simulink model "PFE_2Lignes_RNA (2)"  (R2024a)
settings: Solver=ode4  StartTime=0.0  StopTime=0.18  RelTol=1e-3
libraries: neural x202, spsRMSLib x12, spsThreePhasePISectionLineLib x4, spsThreePhaseFaultLib x2, spsThreePhaseVIMeasurementLib x2, spsThreePhaseSourceLib x2, spspowerguiLib x1
(part 10 of 10)

== system PFE_2Lignes_RNA (2)/RNA_Localisateur/Layer 3/Delays 1 ==
  "p{3}" : Inport  PortDimensions=25
      mask Display: e = 0.06;c1 = [120 230 180]/255;c2 = ([120 230 180]+0)/(256+128);c3 = ([120 230 180]+128)/(256+128);patch([0 1 1 0],[0 0 1 1],c1);patch([0 1 1 1-e 1-e 0+e],[0 0 1 1-e 0+e 0+e],c2);patch([0 0 1 1-e 0+e 0+e],[0 1 1 1-e 1-e 0+e],c3);plot([0 1 1 0 0],[0 0 1 1 0]);
  mux : Mux  Inputs=1
      mask Display: e = 0.06;c1 = [120 150 230]/255;c2 = ([120 150 230]+0)/383;c3 = ([120 150 230]+128)/383;patch([0 1 1 0],[0 0 1 1],c1);patch([0 1 1 1-e 1-e 0+e],[0 0 1 1-e 0+e 0+e],c2);patch([0 0 1 1-e 0+e 0+e],[0 1 1 1-e 1-e 0+e],c3);plot([0 1 1 0 0],[0 0 1 1 0]);disp('Mux')
  "pd{3,2}" : Outport
      mask Display: e = 0.06;c1 = [120 230 180]/255;c2 = ([120 230 180]+0)/(256+128);c3 = ([120 230 180]+128)/(256+128);patch([0 1 1 0],[0 0 1 1],c1);patch([0 1 1 1-e 1-e 0+e],[0 0 1 1-e 0+e 0+e],c2);patch([0 0 1 1-e 0+e 0+e],[0 1 1 1-e 1-e 0+e],c3);plot([0 1 1 0 0],[0 0 1 1 0]);
  wires:
  "p{3}"/1 -> mux/1
  mux/1 -> "pd{3,2}"/1

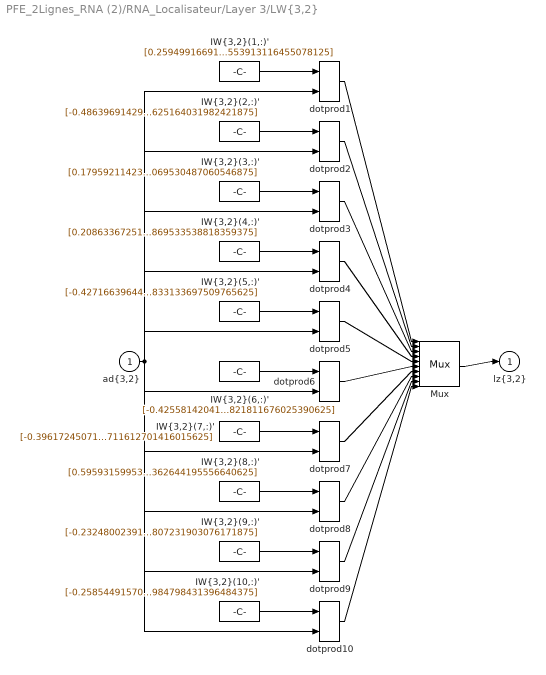
== system PFE_2Lignes_RNA (2)/RNA_Localisateur/Layer 3/LW{3,2} ==
  "ad{3,2}" : Inport  PortDimensions=25
      mask Display: e = 0.06;c1 = [120 230 180]/255;c2 = ([120 230 180]+0)/(256+128);c3 = ([120 230 180]+128)/(256+128);patch([0 1 1 0],[0 0 1 1],c1);patch([0 1 1 1-e 1-e 0+e],[0 0 1 1-e 0+e 0+e],c2);patch([0 0 1 1-e 0+e 0+e],[0 1 1 1-e 1-e 0+e],c3);plot([0 1 1 0 0],[0 0 1 1 0]);
  "IW{3,2}(1,:)'" : Constant  Value=[0.259499166914273715622840654759784229099750518798828125;-0.257383375091483734831143692645127885043621063232421875;-0.0215920617215718847747840669626384624280035495758056640625;-0.38639212006215284400667542286100797355175018310546875;0.0724580935613540477735483591459342278540134429931640625;-0.153650430968274964715902797252056188881397247314453125;-0.5162510887242304224997724304557777941226959228515625;0.0225239402589197008908161734552777488715946674346923828125;-0.330358684113883527277977236735750921070575714111328125;0.169424344213606470344046783793601207435131072998046875;0.07892490230528238781548822089462191797792911529541015625;0.8200359869986921790285805400344543159008026123046875;0.124512774480091514828217214017058722674846649169921875;0.1442480998551381732308840355472057126462459564208984375;-0.53065073451970057316628981425310485064983367919921875;0.2116724722061891217350648730644024908542633056640625;0.16550316479374627132159503162256442010402679443359375;0.396942477917246849816734766136505641043186187744140625;0.033487838311827382298258015680403332225978374481201171875;-0.2078927394991537946911108747372054494917392730712890625;0.24309155258077008721073752894881181418895721435546875;0.2102599726857405648683396748310769908130168914794921875;0.28148895042717192449543972543324343860149383544921875;0.15969935949450875245503311816719360649585723876953125;-0.4549152584406943589101501856930553913116455078125]
      mask Display: e = 0.06;c1 = [120 150 230]/255;c2 = ([120 150 230]+0)/383;c3 = ([120 150 230]+128)/383;patch([0 1 1 0],[0 0 1 1],c1);patch([0 1 1 1-e 1-e 0+e],[0 0 1 1-e 0+e 0+e],c2);patch([0 0 1 1-e 0+e 0+e],[0 1 1 1-e 1-e 0+e],c3);plot([0 1 1 0 0],[0 0 1 1 0]);disp('weights');
  "IW{3,2}(10,:)'" : Constant  Value=[-0.25854491570469650962849073039251379668712615966796875;0.196184940707442134755211782248807139694690704345703125;0.7645250944377817159391952372970990836620330810546875;-0.0184527315099401560682945699909396353177726268768310546875;0.367147579101182841565531589367310516536235809326171875;0.331249780882799382819570155334076844155788421630859375;0.3277245040461982394930373629904352128505706787109375;-0.253855352684368040794282705974183045327663421630859375;0.29341155210540825759579774967278353869915008544921875;0.08151026931019385302068513965423335321247577667236328125;0.1810431757750518844130027673600125126540660858154296875;0.2314159756638828613350966634243377484381198883056640625;0.08787736385978257847018113579906639643013477325439453125;-0.37698257865251705300835283196647651493549346923828125;0.315315557570428506295456827501766383647918701171875;0.33180976505799197884272189185139723122119903564453125;-0.25777939796702875607792293521924875676631927490234375;0.79791774501736811853191966292797587811946868896484375;-0.59432999568261346556852231515222229063510894775390625;-0.61707616054659808479954108406673185527324676513671875;-0.730705022070508025677781915874220430850982666015625;-0.360402877050402137282247849725536070764064788818359375;-0.36782434924704343615076140849851071834564208984375;-0.260230331044378926375060245845816098153591156005859375;-0.27207637131283080034194199470221064984798431396484375]
      mask Display: e = 0.06;c1 = [120 150 230]/255;c2 = ([120 150 230]+0)/383;c3 = ([120 150 230]+128)/383;patch([0 1 1 0],[0 0 1 1],c1);patch([0 1 1 1-e 1-e 0+e],[0 0 1 1-e 0+e 0+e],c2);patch([0 0 1 1-e 0+e 0+e],[0 1 1 1-e 1-e 0+e],c3);plot([0 1 1 0 0],[0 0 1 1 0]);disp('weights');
  "IW{3,2}(2,:)'" : Constant  Value=[-0.486396914294387971988697927372413687407970428466796875;-0.2992436697012557100805452137137763202190399169921875;-1.0096640245988937056864642727305181324481964111328125;-0.7633555721722729003886342979967594146728515625;0.319862500795322912683360527807963080704212188720703125;-0.1381707631856110840562479324944433756172657012939453125;0.05730667196484000303069450410475837998092174530029296875;0.60670341083743528631799790673539973795413970947265625;0.162744168043399473067012195315328426659107208251953125;0.76390045801718053919415751806809566915035247802734375;-0.251036863009820365721935786496032960712909698486328125;0.348548775645059760730504194725654087960720062255859375;-1.2651758025279082886527248774655163288116455078125;0.5701608488095846194454452415811829268932342529296875;-0.45746006806566763547294840464019216597080230712890625;0.1775172818765219096004415177958435378968715667724609375;0.83109712322488393798636252540745772421360015869140625;-0.002819460130945704127991557896848462405614554882049560546875;-1.3113587123974017600858132936991751194000244140625;-0.94794595241073997815561824609176255762577056884765625;-0.8672272284534410236034318586462177336215972900390625;0.31406958478618396402026746727642603218555450439453125;-0.66306336271592503095462234341539442539215087890625;0.70909112904029758528423599273082800209522247314453125;-0.1927834405910741899514704300599987618625164031982421875]
      mask Display: e = 0.06;c1 = [120 150 230]/255;c2 = ([120 150 230]+0)/383;c3 = ([120 150 230]+128)/383;patch([0 1 1 0],[0 0 1 1],c1);patch([0 1 1 1-e 1-e 0+e],[0 0 1 1-e 0+e 0+e],c2);patch([0 0 1 1-e 0+e 0+e],[0 1 1 1-e 1-e 0+e],c3);plot([0 1 1 0 0],[0 0 1 1 0]);disp('weights');
  "IW{3,2}(3,:)'" : Constant  Value=[0.1795921142321371399841467564328922890126705169677734375;-0.0830058214984936981739593875317950733006000518798828125;0.42600710957444254400883210109896026551723480224609375;0.56216901247103800987048316528671421110630035400390625;0.214484010219940568475749387289397418498992919921875;0.65506656139687013951089511465397663414478302001953125;-0.2738986952750577241744167622528038918972015380859375;-0.40274361448586504241831107719917781651020050048828125;0.75469640022346806684794273678562603890895843505859375;0.16066872870166559739146805441123433411121368408203125;0.4675408868247641347437593140057288110256195068359375;0.339255842745214142297527359914965927600860595703125;-0.76204632162776364534551021279185079038143157958984375;0.411196253292331892481570321251638233661651611328125;-0.37118321250245944753487492562271654605865478515625;-0.34219671096980908142626276458031497895717620849609375;-0.26652835547218012290926481000497005879878997802734375;0.46914434545171557200404777177027426660060882568359375;-0.2265549344525312758236168519943021237850189208984375;-0.250327500477882713969535188880399800837039947509765625;-0.5644921592451357383879440021701157093048095703125;-0.02543337437470427619956581111182458698749542236328125;0.215714533272492403614961631319602020084857940673828125;0.133709939839643354719811441100318916141986846923828125;0.45080169671964920308226965062203817069530487060546875]
      mask Display: e = 0.06;c1 = [120 150 230]/255;c2 = ([120 150 230]+0)/383;c3 = ([120 150 230]+128)/383;patch([0 1 1 0],[0 0 1 1],c1);patch([0 1 1 1-e 1-e 0+e],[0 0 1 1-e 0+e 0+e],c2);patch([0 0 1 1-e 0+e 0+e],[0 1 1 1-e 1-e 0+e],c3);plot([0 1 1 0 0],[0 0 1 1 0]);disp('weights');
  "IW{3,2}(4,:)'" : Constant  Value=[0.208633672511950918337930716006667353212833404541015625;-0.049774452361300458580473105030250735580921173095703125;0.439326907042213388177032129533472470939159393310546875;0.171290457666205264697367738335742615163326263427734375;0.540872208754529015806156166945584118366241455078125;-0.2331890730032175340635802740507642738521099090576171875;-0.46194631852841505637030650177621282637119293212890625;0.354039924065002786779388088689302094280719757080078125;0.48242957728458579769181824303814209997653961181640625;0.7025339975202451459068697658949531614780426025390625;-0.471942860262994423603544191792025230824947357177734375;-0.34067847690385588688144480329356156289577484130859375;-0.10191518091187268257868936416343785822391510009765625;0.89719408490654384280560407205484807491302490234375;-0.1476056157321989636965753334152395837008953094482421875;0.371494341788785431557329275165102444589138031005859375;0.53142307222104723241073997996863909065723419189453125;-0.86911676430513173929881531876162625849246978759765625;0.95899584831374007354298782956902869045734405517578125;0.01514824633352983285217163711422472260892391204833984375;-0.0309472140695323354175894081663500401191413402557373046875;0.0227440549634588227989606679102507769130170345306396484375;0.2054332578510936480054027697406127117574214935302734375;0.47578074684271276506564163355506025254726409912109375;-0.493126298182259004132532709263614378869533538818359375]
      mask Display: e = 0.06;c1 = [120 150 230]/255;c2 = ([120 150 230]+0)/383;c3 = ([120 150 230]+128)/383;patch([0 1 1 0],[0 0 1 1],c1);patch([0 1 1 1-e 1-e 0+e],[0 0 1 1-e 0+e 0+e],c2);patch([0 0 1 1-e 0+e 0+e],[0 1 1 1-e 1-e 0+e],c3);plot([0 1 1 0 0],[0 0 1 1 0]);disp('weights');
  "IW{3,2}(5,:)'" : Constant  Value=[-0.42716639644105691697717475108220241963863372802734375;0.319735122611505107048657237100997008383274078369140625;-0.144913256802170875570112684727064333856105804443359375;0.418094711227112558749041681949165649712085723876953125;0.511325541048309961666973322280682623386383056640625;-0.008907182515639870679091671945570851676166057586669921875;-0.289029559077883357876004311037831939756870269775390625;-0.01209733468703781157638221799288658075965940952301025390625;0.039414040601209114622616169754110160283744335174560546875;-0.08724077377198026506111006028731935657560825347900390625;0.93062461612003410937887792897527106106281280517578125;-0.84348086792044563164694181978120468556880950927734375;-0.33012975187102266971805875073187053203582763671875;0.6052379701685082213913347004563547670841217041015625;-0.59579112157312319464352867726120166480541229248046875;0.4111185993323529519472003812552429735660552978515625;0.45409004664972230091990468281437642872333526611328125;0.8687099235218556092519293088116683065891265869140625;0.35767499887355003185263058185228146612644195556640625;-0.59731612138546619217294164627674035727977752685546875;0.162670883357776741018341226663324050605297088623046875;-0.2230248190546767206310363462762325070798397064208984375;-0.573880672304131422833961551077663898468017578125;-0.45711823783840788149035461174207739531993865966796875;0.1625955550529826487693441094961599446833133697509765625]
      mask Display: e = 0.06;c1 = [120 150 230]/255;c2 = ([120 150 230]+0)/383;c3 = ([120 150 230]+128)/383;patch([0 1 1 0],[0 0 1 1],c1);patch([0 1 1 1-e 1-e 0+e],[0 0 1 1-e 0+e 0+e],c2);patch([0 0 1 1-e 0+e 0+e],[0 1 1 1-e 1-e 0+e],c3);plot([0 1 1 0 0],[0 0 1 1 0]);disp('weights');
  "IW{3,2}(6,:)'" : Constant  Value=[-0.425581420418537137440040396541007794439792633056640625;0.11336041614642834718384989400874474085867404937744140625;-0.293111819207529544772938834285014308989048004150390625;0.39126271714747107299814388170489110052585601806640625;0.44854646393908093049418539521866478025913238525390625;0.463505961310431591204661572191980667412281036376953125;-0.397849466360224834904357749110204167664051055908203125;0.284078924760211515287977590560331009328365325927734375;-0.414256591580237032435007904496160335838794708251953125;-0.374072668830715271415243705632747150957584381103515625;0.85195121714305976912129381162230856716632843017578125;0.06469055391895263407153748858036124147474765777587890625;0.85097433591525073470762663419009186327457427978515625;-0.181106906938278466867586757871322333812713623046875;0.34245989875019022807833835031487978994846343994140625;0.646702640754573732095877858228050172328948974609375;-0.5654784119053679614097518424387089908123016357421875;-0.36053840646464208052890398903400637209415435791015625;0.07719239096012538159374827273495611734688282012939453125;-0.28537380618497187878546128558809868991374969482421875;0.54880359654620658460544291301630437374114990234375;0.32469019193151826829790707051870413124561309814453125;0.246685178608404609423843112381291575729846954345703125;-0.2522084322168911540984481689520180225372314453125;0.057301412441833933508750220653382712043821811676025390625]
      mask Display: e = 0.06;c1 = [120 150 230]/255;c2 = ([120 150 230]+0)/383;c3 = ([120 150 230]+128)/383;patch([0 1 1 0],[0 0 1 1],c1);patch([0 1 1 1-e 1-e 0+e],[0 0 1 1-e 0+e 0+e],c2);patch([0 0 1 1-e 0+e 0+e],[0 1 1 1-e 1-e 0+e],c3);plot([0 1 1 0 0],[0 0 1 1 0]);disp('weights');
  "IW{3,2}(7,:)'" : Constant  Value=[-0.3961724507194579469882000921643339097499847412109375;0.1387250010604408612113758181294542737305164337158203125;0.79843909814126001744938321280642412602901458740234375;-0.13197386480330586255860225719516165554523468017578125;-0.963138474221520990425915442756377160549163818359375;0.77614602963594558904247833197587169706821441650390625;0.0459985084465074633985892660348326899111270904541015625;-0.32747154753047247321973145517404191195964813232421875;0.329878955635281745362163974277791567146778106689453125;-0.68783651058276207290731463217525742948055267333984375;1.7187260561734889474649889962165616452693939208984375;0.277645949269099745482236585303326137363910675048828125;-0.0973489866815408222411321048639365471899509429931640625;-1.09730793256456049533653640537522733211517333984375;0.478189280833778929125088552609668113291263580322265625;0.23624340435405011273672926108702085912227630615234375;-0.376796535196192439176599009442725218832492828369140625;0.89917669709510317233025489258579909801483154296875;-0.38151855174703774853384175003156997263431549072265625;-0.243324845860096450333998063797480426728725433349609375;-0.58220435207547371891934062659856863319873809814453125;0.2166088158148688214144073072020546533167362213134765625;0.667135572700811252389030414633452892303466796875;-0.77032076667743165643287284183315932750701904296875;0.036010859707251409445039058709880919195711612701416015625]
      mask Display: e = 0.06;c1 = [120 150 230]/255;c2 = ([120 150 230]+0)/383;c3 = ([120 150 230]+128)/383;patch([0 1 1 0],[0 0 1 1],c1);patch([0 1 1 1-e 1-e 0+e],[0 0 1 1-e 0+e 0+e],c2);patch([0 0 1 1-e 0+e 0+e],[0 1 1 1-e 1-e 0+e],c3);plot([0 1 1 0 0],[0 0 1 1 0]);disp('weights');
  "IW{3,2}(8,:)'" : Constant  Value=[0.5959315995396183840426829192438162863254547119140625;-0.68920983699735038907618900339002721011638641357421875;-0.547275052350105095655408149468712508678436279296875;-0.46668802981562673704019061915460042655467987060546875;0.70348097684159427434025246839155443012714385986328125;1.2358100589287006609851005123346112668514251708984375;-0.057695062285977379012980037487068329937756061553955078125;1.3383434388428316896835212901351042091846466064453125;0.95131380634382989303077238218975253403186798095703125;0.1426293234011531685379026157534099183976650238037109375;-0.54812770381903674898893541467259638011455535888671875;0.7382984438201518617717056258697994053363800048828125;-1.133045117712822236200054248911328613758087158203125;-0.94071248542285046401190129472524859011173248291015625;-0.222026415195621662501679338674875907599925994873046875;0.2989728874563242211337410481064580380916595458984375;0.80555562586803730606987983264843933284282684326171875;-1.630533738843426672104897079407237470149993896484375;-0.9069177750597390286202426068484783172607421875;-0.564683822516274691594162504770793020725250244140625;0.143682760802573195046960563558968715369701385498046875;1.4286546216244477847112648305483162403106689453125;-0.036125095413979291247841274525853805243968963623046875;0.354152440418581349046434070260147564113140106201171875;0.2022263960100302571110120197772630490362644195556640625]
      mask Display: e = 0.06;c1 = [120 150 230]/255;c2 = ([120 150 230]+0)/383;c3 = ([120 150 230]+128)/383;patch([0 1 1 0],[0 0 1 1],c1);patch([0 1 1 1-e 1-e 0+e],[0 0 1 1-e 0+e 0+e],c2);patch([0 0 1 1-e 0+e 0+e],[0 1 1 1-e 1-e 0+e],c3);plot([0 1 1 0 0],[0 0 1 1 0]);disp('weights');
  "IW{3,2}(9,:)'" : Constant  Value=[-0.232480023916576072906536865048110485076904296875;-0.164443579735376654848977295841905288398265838623046875;1.4179787649137292060430581841501407325267791748046875;0.25143330694485344078970001646666787564754486083984375;-0.510136233004576222782588956761173903942108154296875;-0.686297218738918246572211501188576221466064453125;-0.262326282237484331716359520214609801769256591796875;-0.597869214900524692524186320952139794826507568359375;-1.0275285597316126118272450185031630098819732666015625;-0.315286007568047532689803347238921560347080230712890625;0.393766399328244809385779490185086615383625030517578125;-0.5387605194849260925593625870533287525177001953125;-0.006413070897718455010139138039448880590498447418212890625;-0.45177115742190421254775856141350232064723968505859375;0.07537030025988909753831279658697894774377346038818359375;-0.9771504767164269633639150924864225089550018310546875;-0.261093310200134709475605632178485393524169921875;0.481535901719132131137968144685146398842334747314453125;0.570459672953978813580988571629859507083892822265625;0.181741283610712012208665555590414442121982574462890625;-0.79097702615542575532714408836909569799900054931640625;-0.0656079654481984686498208247940056025981903076171875;-0.6737649753269134844657628491404466331005096435546875;0.78476774835336005065045128503697924315929412841796875;-0.078997850155492599366624517642776481807231903076171875]
      mask Display: e = 0.06;c1 = [120 150 230]/255;c2 = ([120 150 230]+0)/383;c3 = ([120 150 230]+128)/383;patch([0 1 1 0],[0 0 1 1],c1);patch([0 1 1 1-e 1-e 0+e],[0 0 1 1-e 0+e 0+e],c2);patch([0 0 1 1-e 0+e 0+e],[0 1 1 1-e 1-e 0+e],c3);plot([0 1 1 0 0],[0 0 1 1 0]);disp('weights');
  Mux : Mux  Inputs=10
      mask Display: e = 0.06;c1 = [120 150 230]/255;c2 = ([120 150 230]+0)/383;c3 = ([120 150 230]+128)/383;patch([0 1 1 0],[0 0 1 1],c1);patch([0 1 1 1-e 1-e 0+e],[0 0 1 1-e 0+e 0+e],c2);patch([0 0 1 1-e 0+e 0+e],[0 1 1 1-e 1-e 0+e],c3);plot([0 1 1 0 0],[0 0 1 1 0]);disp('Mux');
  dotprod{1..10} (10 alike) : neural/Weight Functions/dotprod
  "lz{3,2}" : Outport
      mask Display: e = 0.06;c1 = [120 230 180]/255;c2 = ([120 230 180]+0)/(256+128);c3 = ([120 230 180]+128)/(256+128);patch([0 1 1 0],[0 0 1 1],c1);patch([0 1 1 1-e 1-e 0+e],[0 0 1 1-e 0+e 0+e],c2);patch([0 0 1 1-e 0+e 0+e],[0 1 1 1-e 1-e 0+e],c3);plot([0 1 1 0 0],[0 0 1 1 0]);
  wires:
  "IW{3,2}(1,:)'"/1 -> dotprod1/1
  "ad{3,2}"/1 -> dotprod1/2, dotprod2/2, dotprod3/2, dotprod4/2, dotprod5/2, dotprod6/2, dotprod7/2, dotprod8/2, dotprod9/2, dotprod10/2
  dotprod1/1 -> Mux/1
  "IW{3,2}(2,:)'"/1 -> dotprod2/1
  dotprod2/1 -> Mux/2
  "IW{3,2}(3,:)'"/1 -> dotprod3/1
  dotprod3/1 -> Mux/3
  "IW{3,2}(4,:)'"/1 -> dotprod4/1
  dotprod4/1 -> Mux/4
  "IW{3,2}(5,:)'"/1 -> dotprod5/1
  dotprod5/1 -> Mux/5
  "IW{3,2}(6,:)'"/1 -> dotprod6/1
  dotprod6/1 -> Mux/6
  "IW{3,2}(7,:)'"/1 -> dotprod7/1
  dotprod7/1 -> Mux/7
  "IW{3,2}(8,:)'"/1 -> dotprod8/1
  dotprod8/1 -> Mux/8
  "IW{3,2}(9,:)'"/1 -> dotprod9/1
  dotprod9/1 -> Mux/9
  "IW{3,2}(10,:)'"/1 -> dotprod10/1
  dotprod10/1 -> Mux/10
  Mux/1 -> "lz{3,2}"/1

== system PFE_2Lignes_RNA (2)/RNA_Localisateur/Layer 4/Delays 1 ==
  "p{4}" : Inport  PortDimensions=10
      mask Display: e = 0.06;c1 = [120 230 180]/255;c2 = ([120 230 180]+0)/(256+128);c3 = ([120 230 180]+128)/(256+128);patch([0 1 1 0],[0 0 1 1],c1);patch([0 1 1 1-e 1-e 0+e],[0 0 1 1-e 0+e 0+e],c2);patch([0 0 1 1-e 0+e 0+e],[0 1 1 1-e 1-e 0+e],c3);plot([0 1 1 0 0],[0 0 1 1 0]);
  mux : Mux  Inputs=1
      mask Display: e = 0.06;c1 = [120 150 230]/255;c2 = ([120 150 230]+0)/383;c3 = ([120 150 230]+128)/383;patch([0 1 1 0],[0 0 1 1],c1);patch([0 1 1 1-e 1-e 0+e],[0 0 1 1-e 0+e 0+e],c2);patch([0 0 1 1-e 0+e 0+e],[0 1 1 1-e 1-e 0+e],c3);plot([0 1 1 0 0],[0 0 1 1 0]);disp('Mux')
  "pd{4,3}" : Outport
      mask Display: e = 0.06;c1 = [120 230 180]/255;c2 = ([120 230 180]+0)/(256+128);c3 = ([120 230 180]+128)/(256+128);patch([0 1 1 0],[0 0 1 1],c1);patch([0 1 1 1-e 1-e 0+e],[0 0 1 1-e 0+e 0+e],c2);patch([0 0 1 1-e 0+e 0+e],[0 1 1 1-e 1-e 0+e],c3);plot([0 1 1 0 0],[0 0 1 1 0]);
  wires:
  "p{4}"/1 -> mux/1
  mux/1 -> "pd{4,3}"/1

== system PFE_2Lignes_RNA (2)/RNA_Localisateur/Layer 4/LW{4,3} ==
  "ad{4,3}" : Inport  PortDimensions=10
      mask Display: e = 0.06;c1 = [120 230 180]/255;c2 = ([120 230 180]+0)/(256+128);c3 = ([120 230 180]+128)/(256+128);patch([0 1 1 0],[0 0 1 1],c1);patch([0 1 1 1-e 1-e 0+e],[0 0 1 1-e 0+e 0+e],c2);patch([0 0 1 1-e 0+e 0+e],[0 1 1 1-e 1-e 0+e],c3);plot([0 1 1 0 0],[0 0 1 1 0]);
  "IW{4,3}(1,:)'" : Constant  Value=[-0.908428834390411221733074853545986115932464599609375;-1.69018404210963435474468496977351605892181396484375;-1.136944049877020912475700242794118821620941162109375;-1.135946885605191969403904295177198946475982666015625;-1.1287359278987294519680517623783089220523834228515625;-0.86359320046450649410729738519876264035701751708984375;0.86643282618900452352050933768623508512973785400390625;-2.255647245406937173584083211608231067657470703125;2.569187621419843026160378940403461456298828125;1.1812602730520318505824661770020611584186553955078125]
      mask Display: e = 0.06;c1 = [120 150 230]/255;c2 = ([120 150 230]+0)/383;c3 = ([120 150 230]+128)/383;patch([0 1 1 0],[0 0 1 1],c1);patch([0 1 1 1-e 1-e 0+e],[0 0 1 1-e 0+e 0+e],c2);patch([0 0 1 1-e 0+e 0+e],[0 1 1 1-e 1-e 0+e],c3);plot([0 1 1 0 0],[0 0 1 1 0]);disp('weights');
  Mux : Mux  Inputs=1
      mask Display: e = 0.06;c1 = [120 150 230]/255;c2 = ([120 150 230]+0)/383;c3 = ([120 150 230]+128)/383;patch([0 1 1 0],[0 0 1 1],c1);patch([0 1 1 1-e 1-e 0+e],[0 0 1 1-e 0+e 0+e],c2);patch([0 0 1 1-e 0+e 0+e],[0 1 1 1-e 1-e 0+e],c3);plot([0 1 1 0 0],[0 0 1 1 0]);disp('Mux');
  dotprod1 : neural/Weight Functions/dotprod
  "lz{4,3}" : Outport
      mask Display: e = 0.06;c1 = [120 230 180]/255;c2 = ([120 230 180]+0)/(256+128);c3 = ([120 230 180]+128)/(256+128);patch([0 1 1 0],[0 0 1 1],c1);patch([0 1 1 1-e 1-e 0+e],[0 0 1 1-e 0+e 0+e],c2);patch([0 0 1 1-e 0+e 0+e],[0 1 1 1-e 1-e 0+e],c3);plot([0 1 1 0 0],[0 0 1 1 0]);
  wires:
  "IW{4,3}(1,:)'"/1 -> dotprod1/1
  "ad{4,3}"/1 -> dotprod1/2
  dotprod1/1 -> Mux/1
  Mux/1 -> "lz{4,3}"/1

== matlab function PFE_2Lignes_RNA (2)/Detecteur ==
  data: u input; y output
function y = Decision_Detecteur(u)

[~,idx] = max(u);

if idx == 1
    y = 0;   % Non défaut
else
    y = 1;   % Défaut
end

== matlab function PFE_2Lignes_RNA (2)/Classificateur ==
  data: u input; classe output
function classe = Decision_Classificateur(u)

[~,classe] = max(u);

% 1 = AG
% 2 = BG
% 3 = CG
% 4 = AB
% 5 = BC
% 6 = AC
% 7 = ABG
% 8 = BCG
% 9 = ACG
% 10 = ABCfunction y = fcn(u)

y = u;
